simulink model "ConfiguredVirtualVehicleModel"  (R2024b)
settings: configuration reference "VehicleVariable" (kept outside this file)
InitFcn:
  | % 1. 获取当前路径
  | current_path = pwd;
  | 
  | % 2. 找到 "EV" 文件夹所在的位置
  | % 使用文件分隔符切割路径
  | path_parts = strsplit(current_path, filesep);
  | % 找到 'EV' 的索引（如果有多个 EV 文件夹，取最后一个）
  | idx = find(strcmp(path_parts, 'EV'), 1, 'last');
  | 
  | if ~isempty(idx)
  |     % 3. 重组出项目根目录 (D:\GraduationProject\EV)
  |     root_path = strjoin(path_parts(1:idx), filesep);
  | 
  |     % 4. 拼接 Scripts 路径并添加
  |     target_script_path = fullfile(root_path, 'Scripts');
  |     addpath(target_script_path);
  | 
  |     % 可选：顺便把根目录也加进去
  |     addpath(root_path);
  | 
  |     fprintf('>>> 项目环境初始化成功，Script路径已锁定: %s\n', target_script_path);
  | else
  |     warning('无法定位 "EV" 项目根目录，请手动添加 Scripts 路径。');
  | end
StopFcn:
  | % 仿真结束后，自动调用清洗脚本
  | %analyze_results(out);
  | analyze_sim_results(out)
model workspace (MAT data in the model file):
  ExtDrvCmdsSwitch : Simulink.Parameter (value not decoded)
  ExtDrvRefSwitch : Simulink.Parameter (value not decoded)
  ExtEnvSwitch : Simulink.Parameter (value not decoded)
  ExtGndSwitch : Simulink.Parameter (value not decoded)
symbols that are objects in the model workspace (value not decoded): ExtDrvCmdsSwitch, ExtDrvRefSwitch, ExtEnvSwitch, ExtGndSwitch
undefined symbols (not defined in the file or in its folder): AccelCmd, AmbTemp, BaroPress, CurvGradRef, CurvRef, DCM, DecelCmd, DiscIntNeverNeededParam, DriverAeroRes, DriverDrivelineRes, DriverInitialGear, DriverPreviewDist, DriverRollRes, DriverShiftTime, DriverTimeConst, DriverTractiveForce, EnvAbsPrs, EnvAirTemp, EnvGrvty, EnvNomFrictionScaling, EnvNominalGrade, EnvWindVelX, EnvWindVelY, EnvWindVelZ, Gnd, Grade, HazzardCmd, HighBeamCmd, lambda_mux, LeftSignalCmd, LngRef, Location, LowBeamCmd, LtrRef, Orientation, PhiRef, PlntVehDstCGFrntAxl, PlntVehDstCGRearAxl, PlntVehInitLatPos, PlntVehInitLongPos, PlntVehInitPitchAng, PlntVehInitRollAng, PlntVehInitVertPos, PlntVehInitYawAng, PlntVehMass, PlntVehTrckWdth, PlntVehYawMomentInertia, PlntWhlLdRadiusFrnt, PlntWhlLdRadiusRear, RightSignalCmd, ScnCRRadius, Sim3dSensor, SteerCmd, Wind, XRef, YRef, Z
libraries: simulink x27, autolibutils x8, autolibsharedcommon x7, vehdynlibscenariocommon x7, vehdynlibviscommon x4, sim3dautolib x4, vrlib x2, vehdynlibdriver x2, sim3dgroundtruthsensorlib x2, autolibshared x2, sharedtransform x1, drivingscenarioandsensors x1
(part 6 of 6)

== system ConfiguredVirtualVehicleModel/Visualization/3D Engine/3D Engine/Scale/PartConcatenation ==
  BodyX : Inport
  BodyY : Inport  Port=2
  BodyZ : Inport  Port=3
  WheelFrontLeftX : Inport  Port=4
  WheelFrontLeftY : Inport  Port=5
  WheelFrontLeftZ : Inport  Port=6
  WheelFrontRightX : Inport  Port=7
  WheelFrontRightY : Inport  Port=8
  WheelFrontRightZ : Inport  Port=9
  WheelRearLeftX : Inport  Port=10
  WheelRearLeftY : Inport  Port=11
  WheelRearLeftZ : Inport  Port=12
  WheelRearRightX : Inport  Port=13
  WheelRearRightY : Inport  Port=14
  WheelRearRightZ : Inport  Port=15
  AllParts : Concatenate  NumInputs=5  Mode=Multidimensional array
  Body : Concatenate  NumInputs=3  Mode=Multidimensional array  ConcatenateDimension=2
  WheelFrontLeft : Concatenate  NumInputs=3  Mode=Multidimensional array  ConcatenateDimension=2
  WheelFrontRight : Concatenate  NumInputs=3  Mode=Multidimensional array  ConcatenateDimension=2
  WheelRearLeft : Concatenate  NumInputs=3  Mode=Multidimensional array  ConcatenateDimension=2
  WheelRearRight : Concatenate  NumInputs=3  Mode=Multidimensional array  ConcatenateDimension=2
  ConcatOut : Outport  VectorParamsAs1DForOutWhenUnconnected=off
  wires:
  WheelFrontRightZ/1 -> WheelFrontRight/3
  WheelRearLeftX/1 -> WheelRearLeft/1
  WheelRearRight/1 -> AllParts/5
  WheelRearLeftY/1 -> WheelRearLeft/2
  AllParts/1 -> ConcatOut/1
  WheelRearLeftZ/1 -> WheelRearLeft/3
  WheelRearRightY/1 -> WheelRearRight/2
  WheelFrontRightX/1 -> WheelFrontRight/1
  WheelFrontRightY/1 -> WheelFrontRight/2
  WheelRearRightZ/1 -> WheelRearRight/3
  WheelFrontRight/1 -> AllParts/3
  WheelRearLeft/1 -> AllParts/4
  Body/1 -> AllParts/1
  WheelRearRightX/1 -> WheelRearRight/1
  WheelFrontLeft/1 -> AllParts/2
  BodyY/1 -> Body/2
  WheelFrontLeftY/1 -> WheelFrontLeft/2
  WheelFrontLeftZ/1 -> WheelFrontLeft/3
  WheelFrontLeftX/1 -> WheelFrontLeft/1
  BodyZ/1 -> Body/3
  BodyX/1 -> Body/1

== system ConfiguredVirtualVehicleModel/Visualization/3D Engine/3D Engine/Trailer/No Trailer ==
  VehFdbk : Inport
  Terminator : Terminator
  wires:
  VehFdbk/1 -> Terminator/1

== system ConfiguredVirtualVehicleModel/Visualization/3D Engine/3D Engine/Trailer/One-Axle Trailer ==
  VehFdbk : Inport
  Simulation 3D Trailer : sim3dautolib/Simulation 3D Trailer  Priority=-1  Mesh=One-axle trailer  ActorName=SimulinkVehicle2  Translation=[PlntVehInitLongPos PlntVehInitLatPos -PlntVehInitVertPos; 0 0 0; 0 0 0]  Rotation=[PlntVehInitRollAng PlntVehInitPitchAng PlntVehInitYawAng; 0 0 0; 0 0 0]  SampleTime=-1  ActorType=SimulinkVehicle  ID=2  aMode=2  ActorTag=SimulinkVehicle2
      settings: LibrarySourceBlock=vehdynlibsim3d/Simulation 3D Trailer
  Trailer Rotation : Subsystem
  Trailer Translation : Subsystem
  wires:
  VehFdbk/1 -> Trailer Translation/1(Trailer), Trailer Rotation/1(Trailer)
  Trailer Rotation/1(Rotation) -> Simulation 3D Trailer/2
  Trailer Translation/1(Translation) -> Simulation 3D Trailer/1

== system ConfiguredVirtualVehicleModel/Environment/Ground Feedback/3D Engine/3D Engine Source/Multiple Points/For Each Subsystem ==
  phi,theta,psi : Inport  Partition=on  PartitionDimension=2  PartitionWidth=1  PartitionOffset=0
  For Each : ForEach  DisableCoverage=on
  Rotation Angles to Direction Cosine Matrix1 : sharedtransform/Rotation Angles to Direction Cosine Matrix  rotationOrder=YXZ  aMode=2
  Selector5 : Selector  InputPortWidth=3  IndexOptions=Index vector (dialog)  Indices=[2 1 3]  OutputSizes=1
  WheelDCM : Outport  ConcatenationDimension=3
  wires:
  Selector5/1 -> Rotation Angles to Direction Cosine Matrix1/1
  Rotation Angles to Direction Cosine Matrix1/1 -> WheelDCM/1
  phi,theta,psi/1 -> Selector5/1

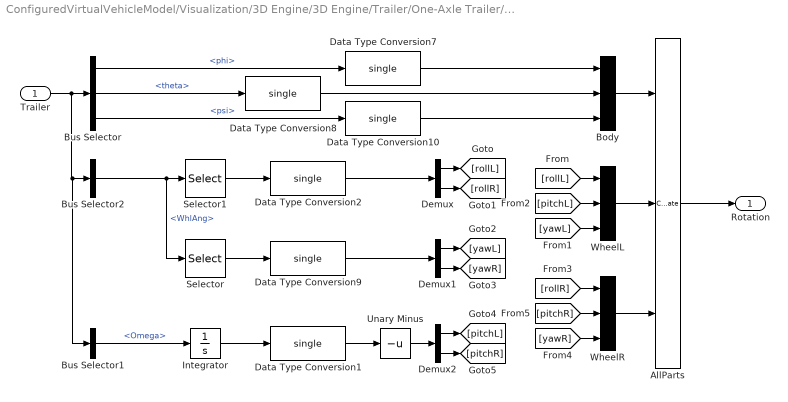
== system ConfiguredVirtualVehicleModel/Visualization/3D Engine/3D Engine/Trailer/One-Axle Trailer/Trailer Rotation ==
  Trailer : Inport
  AllParts : Concatenate  NumInputs=3  Mode=Multidimensional array
  Body : Concatenate  NumInputs=3  Mode=Multidimensional array  ConcatenateDimension=2
  Bus Selector : BusSelector  OutputSignals=TrlrBody.InertFrm.Cg.Ang.phi,TrlrBody.InertFrm.Cg.Ang.theta,TrlrBody.InertFrm.Cg.Ang.psi
  Bus Selector1 : BusSelector  OutputSignals=TrlrWheels.Wheels.TireFrame.Omega
  Bus Selector2 : BusSelector  OutputSignals=TrlrBody.Suspension.WhlAng
  Data Type Conversion{1..2,7..10} (6 alike) : DataTypeConversion  OutDataTypeStr=single  SaturateOnIntegerOverflow=off  RndMeth=Floor
  Demux : Demux  Outputs=2
  Demux1 : Demux  Outputs=2
  Demux2 : Demux  Outputs=2
  Integrator : Integrator  WrapState=on  WrappedStateUpperValue=2*pi  WrappedStateLowerValue=0  ZeroCross=off
  Selector : Selector  NumberOfDimensions=2  InputPortWidth=3  IndexOptions=Index vector (dialog),Select all  Indices=[3],1  OutputSizes=1,1
  Selector1 : Selector  NumberOfDimensions=2  InputPortWidth=3  IndexOptions=Index vector (dialog),Select all  Indices=[1],1  OutputSizes=1,1
  Unary Minus : UnaryMinus
  WheelL : Concatenate  NumInputs=3  Mode=Multidimensional array  ConcatenateDimension=2
  WheelR : Concatenate  NumInputs=3  Mode=Multidimensional array  ConcatenateDimension=2
  Rotation : Outport
  wires:
  Trailer/1 -> Bus Selector1/1, Bus Selector2/1, Bus Selector/1
  Body/1 -> AllParts/1
  Bus Selector/1 -> Data Type Conversion7/1  "<phi>"
  Bus Selector/3 -> Data Type Conversion10/1  "<psi>"
  Bus Selector/2 -> Data Type Conversion8/1  "<theta>"
  Selector/1 -> Data Type Conversion9/1
  Data Type Conversion9/1 -> Demux1/1
  Data Type Conversion2/1 -> Demux/1
  Selector1/1 -> Data Type Conversion2/1
  Bus Selector2/1 -> Selector1/1, Selector/1  "<WhlAng>"
  Bus Selector1/1 -> Integrator/1  "<Omega>"
  Integrator/1 -> Data Type Conversion1/1
  Unary Minus/1 -> Demux2/1
  Data Type Conversion1/1 -> Unary Minus/1
  Demux/1 -> [rollL]
  Demux/2 -> [rollR]
  Demux1/2 -> [yawR]
  Demux1/1 -> [yawL]
  Demux2/2 -> [pitchR]
  Demux2/1 -> [pitchL]
  [rollL] -> WheelL/1
  [yawL] -> WheelL/3
  [pitchL] -> WheelL/2
  [rollR] -> WheelR/1
  [yawR] -> WheelR/3
  [pitchR] -> WheelR/2
  WheelR/1 -> AllParts/3
  WheelL/1 -> AllParts/2
  AllParts/1 -> Rotation/1
  Data Type Conversion7/1 -> Body/1
  Data Type Conversion8/1 -> Body/2
  Data Type Conversion10/1 -> Body/3

== system ConfiguredVirtualVehicleModel/Visualization/3D Engine/3D Engine/Trailer/One-Axle Trailer/Trailer Translation ==
  Trailer : Inport
  AllParts : Concatenate  NumInputs=3  Mode=Multidimensional array
  Body : Concatenate  NumInputs=3  Mode=Multidimensional array  ConcatenateDimension=2
  Bus Selector : BusSelector  OutputSignals=TrlrBody.InertFrm.HitchF.Disp.X,TrlrBody.InertFrm.HitchF.Disp.Y,TrlrBody.InertFrm.Cg.Disp.Z
  Bus Selector1 : BusSelector  OutputSignals=TrlrBody.Suspension.dz
  Constant : Constant  Value=0  OutDataTypeStr=single
  Constant1 : Constant  Value=0  OutDataTypeStr=single
  Data Type Conversion{1,7..8,10} (4 alike) : DataTypeConversion  OutDataTypeStr=single  SaturateOnIntegerOverflow=off  RndMeth=Floor
  Demux : Demux  Outputs=2
  Unary Minus1 : UnaryMinus
  WheelL : Concatenate  NumInputs=3  Mode=Multidimensional array  ConcatenateDimension=2
  WheelR : Concatenate  NumInputs=3  Mode=Multidimensional array  ConcatenateDimension=2
  Translation : Outport
  wires:
  Trailer/1 -> Bus Selector1/1, Bus Selector/1
  Bus Selector/1 -> Data Type Conversion7/1  "<X>"
  Bus Selector/2 -> Data Type Conversion8/1  "<Y>"
  Bus Selector/3 -> Data Type Conversion10/1  "<Z>"
  Data Type Conversion7/1 -> Body/1
  Data Type Conversion8/1 -> Body/2
  Data Type Conversion10/1 -> Body/3
  Unary Minus1/1 -> Demux/1
  Bus Selector1/1 -> Data Type Conversion1/1  "<dz>"
  WheelL/1 -> AllParts/2
  Body/1 -> AllParts/1
  AllParts/1 -> Translation/1
  WheelR/1 -> AllParts/3
  Demux/1 -> [zL]
  Demux/2 -> [zR]
  [zR] -> WheelR/3
  [zL] -> WheelL/3
  Constant/1 -> WheelL/2, WheelL/1
  Constant1/1 -> WheelR/2, WheelR/1
  Data Type Conversion1/1 -> Unary Minus1/1

== stateflow chart ConfiguredVirtualVehicleModel/Driver Commands/Subsystem/Chart ==
  state Auto_Active
    entry: isAuto = 1;
  state Manual
    entry: isAuto = 0;
  (default) -> Manual
  Manual -> Auto_Active : [btnRise == 1 && Driver_Brake < 0.05 && Driver_Accel < 0.05 && abs(Driver_Steer) < 0.05]
  Auto_Active -> Manual [order 1] : [btnRise == 1]
  Auto_Active -> Manual [order 2] : [Driver_Brake > 0.05 || Driver_Accel > 0.05 || abs(Driver_Steer) > 0.05]
  data: ChartMode output Enum: ChartModeType; isAuto output; btnRise input; Driver_Brake input; Driver_Accel input; Driver_Steer input

== matlab function ConfiguredVirtualVehicleModel/Visualization/3D Engine/3D Engine/MATLAB Function ==
  data: t input; v_lead output; caseID input; y_lead output; yaw_lead output
function [v_lead, y_lead, yaw_lead] = LeadProfile(t, caseID)
% LeadProfile
% 输入:
%   t      - 仿真时间(s), 由 Clock 提供
%   caseID - 工况编号 (1~6)
% 输出:
%   v_lead   - 前车纵向速度(m/s)
%   y_lead   - 前车横向位置(m)
%   yaw_lead - 前车航向角(deg)
%
% 约束:
%   最大速度 20 m/s, 最小速度 0 m/s
%
% 工况定义:
%   1: 匀速20
%   2: 缓刹 20->12
%   3: 急刹 20->0
%   4: Stop&Go
%   5: Cut-in（旁车道切入）
%   6: 综合工况（一次仿真内包含多种典型情况）

vmax = 20;

% 默认值
v_lead = 20;
y_lead = 0;
yaw_lead = 0;   % 先简化为0，直道/轻横向工况够用

switch int32(caseID)

    case 1  % 匀速20
        v_lead = 20;
        y_lead = 0;

    case 2  % 缓刹: 10~18s 从20降到12
        if t < 10
            v_lead = 20;
        elseif t < 18
            v_lead = 20 - (8/8)*(t-10);   % 每秒降1
        else
            v_lead = 12;
        end
        y_lead = 0;

    case 3  % 急刹: 10~12s 从20降到0
        if t < 10
            v_lead = 20;
        elseif t < 12
            v_lead = 20 - 10*(t-10);
        else
            v_lead = 0;
        end
        y_lead = 0;

    case 4  % Stop&Go
        % 0-8:20, 8-12:减到0, 12-20:停, 20-26:加到16, 26+:16
        if t < 8
            v_lead = 20;
        elseif t < 12
            v_lead = 20 - 5*(t-8);
        elseif t < 20
            v_lead = 0;
        elseif t < 26
            v_lead = (16/6)*(t-20);
        else
            v_lead = 16;
        end
        y_lead = 0;

    case 5  % Cut-in: 纵向18，12~18s 横向3.5->0
        v_lead = 18;
        if t < 12
            y_lead = 3.5;  % 相邻车道
        elseif t < 18
            s = (t-12)/6;  % 0~1
            y_lead = 3.5*(1 - (3*s^2 - 2*s^3)); % 平滑切入
        else
            y_lead = 0;
        end

    case 6  % 综合工况（60s内）
        % 0-8: 匀速20
        % 8-16: 缓刹20->12
        % 16-22: 保持12
        % 22-24: 急刹12->0
        % 24-30: 停车
        % 30-36: 起步0->16
        % 36-60: 巡航16
        if t < 8
            v_lead = 20;
        elseif t < 16
            v_lead = 20 - (8/8)*(t-8);
        elseif t < 22
            v_lead = 12;
        elseif t < 24
            v_lead = 12 - 6*(t-22);
        elseif t < 30
            v_lead = 0;
        elseif t < 36
            v_lead = (16/6)*(t-30);
        else
            v_lead = 16;
        end

        % 40-48s 做一次切入: y 3.5 -> 0
        if t < 40
            y_lead = 3.5;
        elseif t < 48
            s = (t-40)/8;  % 0~1
            y_lead = 3.5*(1 - (3*s^2 - 2*s^3));
        else
            y_lead = 0;
        end

    otherwise
        % 默认回到 case1
        v_lead = 20;
        y_lead = 0;
end

% 速度限幅
v_lead = min(max(v_lead,0),vmax);
